simulink model "test_diode_lcl"  (R2021a)
settings: Solver=VariableStepAuto  StartTime=0.0  StopTime=0.2  RelTol=1e-3
values from neighbouring files (symbols this model uses):
  amplitude = 400    [init_diode_3l.m]
  C_dc = 10e-3    (= 0.01)    [init_diode_3l.m]
  C_f = 1e-5    (= 1e-05)    [init_diode_3l.m]
  freq = 50    [init_diode_3l.m]
  L_conv = 100e-5    (= 0.001)    [init_diode_3l.m]
  L_dc = 100e-5    (= 0.001)    [init_diode_3l.m]
  L_dc_src = 100e-1    (= 10)    [init_diode_3l.m]
  L_grid = 100e-5    (= 0.001)    [init_diode_3l.m]
  L_src = 100e-5    (= 0.001)    [init_diode_3l.m]
  R_conv = 1e-3    (= 0.001)    [init_diode_3l.m]
  R_dc = 1e-3    (= 0.001)    [init_diode_3l.m]
  R_dc_p = 100    [init_diode_3l.m]
  R_dc_src = 10    [init_diode_3l.m]
  R_f = 1e-3    (= 0.001)    [init_diode_3l.m]
  R_grid = 1e-3    (= 0.001)    [init_diode_3l.m]
  R_src = 1e-3    (= 0.001)    [init_diode_3l.m]
  V_dc_src = 500    [init_diode_3l.m]
libraries: spsSeriesRLCBranchLib x12, spsThreePhaseSeriesRLCBranchLib x8, spsDiodeLib x6, spsMultimeterLib x1, spsThreePhaseSourceLib x1, spsDCVoltageSourceLib x1, spspowerguiLib x1, spsVoltageMeasurementLib x1
settings Model: Creator=viliv  LastModifiedBy=viliv

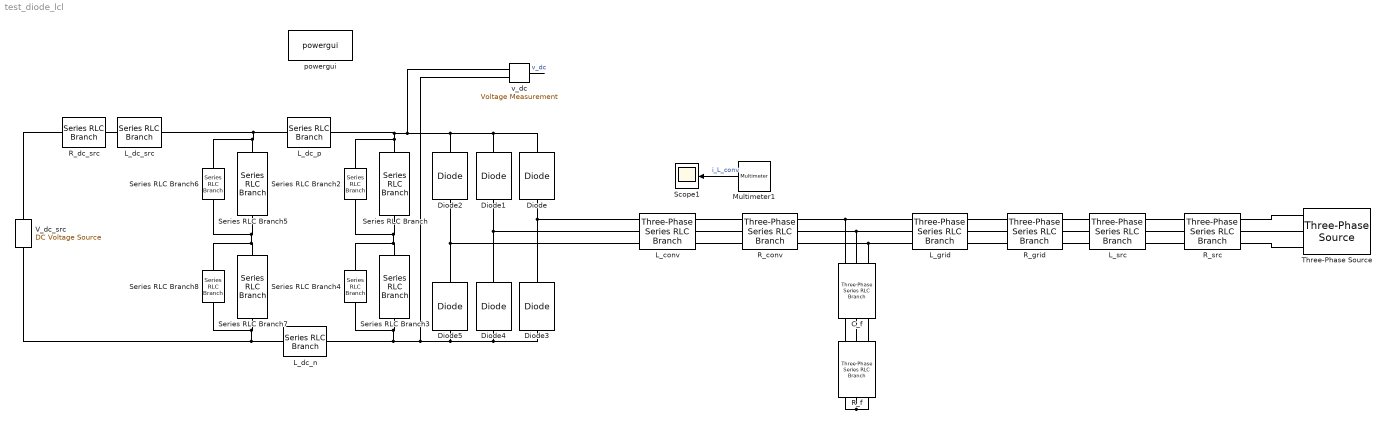
== system test_diode_lcl ==
  C_f : spsThreePhaseSeriesRLCBranchLib/Three-Phase Series RLC Branch  LConnTagsString=A|B|C  RConnTagsString=A|B|C  BranchType=C  Resistance=1  Inductance=100e-6  Capacitance=C_f  Measurements=Branch currents
  Diode{,1..5} (6 alike) : spsDiodeLib/Diode  Ron=1e-8  Lon=0  Vf=0.8  IC=0  UseSnubber=0  Rs=1e6  Cs=250e-12  Measurements=off
  L_conv : spsThreePhaseSeriesRLCBranchLib/Three-Phase Series RLC Branch  LConnTagsString=A|B|C  RConnTagsString=A|B|C  BranchType=L  Resistance=1  Inductance=L_conv  Capacitance=1e-6  Measurements=Branch currents
  L_dc_n : spsSeriesRLCBranchLib/Series RLC Branch  LConnTagsString=__new0  RConnTagsString=__new0  BranchType=L  Resistance=1  Inductance=L_dc  SetiL0=off  InitialCurrent=0  Capacitance=0.05  Setx0=off  InitialVoltage=0  Measurements=None
  L_dc_p : spsSeriesRLCBranchLib/Series RLC Branch  LConnTagsString=__new0  RConnTagsString=__new0  BranchType=L  Resistance=1  Inductance=L_dc  SetiL0=off  InitialCurrent=0  Capacitance=0.05  Setx0=off  InitialVoltage=0  Measurements=None
  L_dc_src : spsSeriesRLCBranchLib/Series RLC Branch  LConnTagsString=__new0  RConnTagsString=__new0  BranchType=L  Resistance=1  Inductance=L_dc_src  SetiL0=off  InitialCurrent=0  Capacitance=0.05  Setx0=off  InitialVoltage=0  Measurements=None
  L_grid : spsThreePhaseSeriesRLCBranchLib/Three-Phase Series RLC Branch  LConnTagsString=A|B|C  RConnTagsString=A|B|C  BranchType=L  Resistance=1  Inductance=L_grid  Capacitance=1e-6  Measurements=Branch currents
  L_src : spsThreePhaseSeriesRLCBranchLib/Three-Phase Series RLC Branch  LConnTagsString=A|B|C  RConnTagsString=A|B|C  BranchType=L  Resistance=1  Inductance=L_src  Capacitance=1e-6  Measurements=Branch currents
  Multimeter1 : spsMultimeterLib/Multimeter  PhasorSimulation=off  OutputType=Complex  sel=[24 25 26]  L=44  Gain=[1 1 1]  yselected={'Ib1: L_conv','Ib2: L_conv','Ib3: L_conv'};  PSBOutputType=1  PSBequivalent=0  AxesSetting=[0,0.1,-100,100]  Display=0  SavedBlockNames=-11
  R_conv : spsThreePhaseSeriesRLCBranchLib/Three-Phase Series RLC Branch  LConnTagsString=A|B|C  RConnTagsString=A|B|C  BranchType=R  Resistance=R_conv  Inductance=0.1  Capacitance=1e-6  Measurements=Branch voltages and currents
  R_dc_src : spsSeriesRLCBranchLib/Series RLC Branch  LConnTagsString=__new0  RConnTagsString=__new0  BranchType=R  Resistance=R_dc_src  Inductance=L_dc  SetiL0=off  InitialCurrent=0  Capacitance=0.05  Setx0=off  InitialVoltage=0  Measurements=None
  R_f : spsThreePhaseSeriesRLCBranchLib/Three-Phase Series RLC Branch  LConnTagsString=A|B|C  RConnTagsString=A|B|C  BranchType=R  Resistance=R_f  Inductance=0.1  Capacitance=1e-6  Measurements=Branch voltages and currents
  R_grid : spsThreePhaseSeriesRLCBranchLib/Three-Phase Series RLC Branch  LConnTagsString=A|B|C  RConnTagsString=A|B|C  BranchType=R  Resistance=R_grid  Inductance=0.1  Capacitance=1e-6  Measurements=Branch voltages and currents
  R_src : spsThreePhaseSeriesRLCBranchLib/Three-Phase Series RLC Branch  LConnTagsString=A|B|C  RConnTagsString=A|B|C  BranchType=R  Resistance=R_src  Inductance=0.1  Capacitance=1e-6  Measurements=Branch voltages and currents
  Scope1 : Scope
  Series RLC Branch{,3,5,7} (4 alike) : spsSeriesRLCBranchLib/Series RLC Branch  LConnTagsString=__new0  RConnTagsString=__new0  BranchType=RC  Resistance=R_dc  Inductance=1e-3  SetiL0=off  InitialCurrent=0  Capacitance=C_dc  Setx0=off  InitialVoltage=0  Measurements=Branch voltage
  Series RLC Branch{2,4,6,8} (4 alike) : spsSeriesRLCBranchLib/Series RLC Branch  LConnTagsString=__new0  RConnTagsString=__new0  BranchType=R  Resistance=R_dc_p  Inductance=1e-3  SetiL0=off  InitialCurrent=0  Capacitance=10e-3  Setx0=off  InitialVoltage=0  Measurements=Branch voltage
  Three-Phase Source : spsThreePhaseSourceLib/Three-Phase Source  InternalConnection=Y  VoltagePhases=off  Voltage=amplitude * sqrt(3) / sqrt(2)  PhaseAngle=initial_angle  Voltage_phases=[25e3 25e3 25e3]/sqrt(3)  PhaseAngles_phases=[0 -120 +120]  Frequency=freq  NonIdealSource=off  SpecifyImpedance=off  Resistance=0.8929  Inductance=16.58e-3  ShortCircuitLevel=100e6  BaseVoltage=25e3  XRratio=7  BusType=swing  Pref=10e3  Qref=0  Prefabc=[10e3, 10e3, 10e3]  Qrefabc=[0, 0, 0]  Qmin=-inf  Qmax=inf
  V_dc_src : spsDCVoltageSourceLib/DC Voltage Source  Amplitude=V_dc_src  Measurements=None
  powergui : spspowerguiLib/powergui  Priority=1  SimulationMode=Discrete  SampleTime=10e-6  frequency=60  Iterations=50  frequencyindice=50  Pbase=100e6  ErrMax=1e-4  UnitsV=kV  UnitsW=MW  buscounter=0  FunctionMessages=off  echomessages=off  EnableUseOfTLC=off  CurrentSourceSwitches=off  DisableSnubberDevices=off  DisableRonSwitches=off  DisableVfSwitches=off  DisplayEquations=off  AutomaticDiscreteSolvers=off  SolverType=Tustin/Backward Euler (TBE)  Interpol=off  ExternalGateDelay=off  methode=off  Ts=100  x0status=zero  SPID=on  SwTol=0  HookPort=off  NonlinearTolerance=1e-4  nMaxIteration=100  ContinueOnMaxIteration=off  RestoreLinks=warning  ResistiveCurrentMeasurement=off  Frange=[0:2:500]  Ylog=off  Xlog=on  ShowGrid=off  save=off  variable=ZData  structure=0  ZoomFFT=off  StartTime=0.0  cycles=1  DisplayStyle=1  fundamental=60  FreqAxis=off  MaxFrequency=1000  frequencyindicesteady=1  RmsSteady=1  display=off
  v_dc : spsVoltageMeasurementLib/Voltage Measurement  PhasorSimulation=off  OutputType=Complex  PSBequivalent=0
  wires:
  Multimeter1/1 -> Scope1/1  "i_L_conv"
  v_dc/1 -> ?  "v_dc"
  connections:
  L_conv/LConn1 -- R_conv/RConn1
  L_conv/LConn2 -- R_conv/RConn2
  L_conv/LConn3 -- R_conv/RConn3
  L_conv/RConn2 -- Diode1/LConn1 -- Diode4/RConn1
  Diode/LConn1 -- Diode3/RConn1 -- L_conv/RConn1
  L_conv/RConn3 -- Diode2/LConn1 -- Diode5/RConn1
  Series RLC Branch5/LConn1 -- L_dc_src/RConn1 -- L_dc_p/LConn1 -- Series RLC Branch6/LConn1
  R_src/LConn2 -- Three-Phase Source/RConn2
  R_src/LConn1 -- Three-Phase Source/RConn1
  R_src/LConn3 -- Three-Phase Source/RConn3
  L_src/LConn1 -- R_src/RConn1
  L_src/LConn2 -- R_src/RConn2
  L_src/LConn3 -- R_src/RConn3
  L_grid/LConn2 -- R_grid/RConn2
  L_grid/LConn3 -- R_grid/RConn3
  L_grid/LConn1 -- R_grid/RConn1
  R_grid/LConn1 -- L_src/RConn1
  R_grid/LConn2 -- L_src/RConn2
  R_grid/LConn3 -- L_src/RConn3
  C_f/RConn2 -- R_f/LConn2
  C_f/RConn1 -- R_f/LConn1
  C_f/RConn3 -- R_f/LConn3
  R_conv/LConn1 -- C_f/LConn1 -- L_grid/RConn1
  R_conv/LConn2 -- L_grid/RConn2 -- C_f/LConn2
  R_conv/LConn3 -- L_grid/RConn3 -- C_f/LConn3
  R_f/RConn1 -- R_f/RConn2 -- R_f/RConn3
  Series RLC Branch/RConn1 -- Series RLC Branch3/LConn1 -- Series RLC Branch4/LConn1 -- Series RLC Branch2/RConn1
  Diode3/LConn1 -- v_dc/LConn2 -- L_dc_n/RConn1 -- Series RLC Branch3/RConn1 -- Series RLC Branch4/RConn1 -- Diode5/LConn1 -- Diode4/LConn1
  Series RLC Branch8/LConn1 -- Series RLC Branch6/RConn1 -- Series RLC Branch5/RConn1 -- Series RLC Branch7/LConn1
  Series RLC Branch2/LConn1 -- L_dc_p/RConn1 -- v_dc/LConn1 -- Diode/RConn1 -- Diode1/RConn1 -- Diode2/RConn1 -- Series RLC Branch/LConn1
  R_dc_src/RConn1 -- L_dc_src/LConn1
  V_dc_src/RConn1 -- R_dc_src/LConn1
  Series RLC Branch8/RConn1 -- V_dc_src/LConn1 -- L_dc_n/LConn1 -- Series RLC Branch7/RConn1
